simulink model "bloco_Main"  (R2015a)
settings: Solver=ode45  StartTime=0.0  StopTime=10.0  RelTol=1e-3
settings Model: Creator=YecidMoreno  LastModifiedBy=YecidMoreno

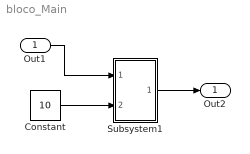
== system bloco_Main ==
  Out1 : Inport
  Constant : Constant  Value=10
  Subsystem1 : Subsystem
  Out2 : Outport
  wires:
  Constant/1 -> Subsystem1/2(In2)
  Subsystem1/1(Out1) -> Out2/1
  Out1/1 -> Subsystem1/1(In1)

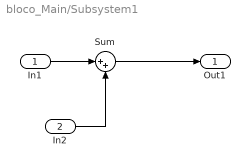
== system bloco_Main/Subsystem1 ==
  In1 : Inport
  In2 : Inport  Port=2
  Sum : Sum  Inputs=|++
  Out1 : Outport
  wires:
  Sum/1 -> Out1/1
  In1/1 -> Sum/1
  In2/1 -> Sum/2
